simulink model "EKF_SPM_Slx2019"  (R2019a)
settings: Solver=ode45  StartTime=0.0  StopTime=0.7  MaxStep=5e-6  RelTol=1e-3
values from neighbouring files (symbols this model uses):
  alpha = 2*pi*200    (= 1256.63706144)    [EKF_SPM_settings.m]
  alphas = log(9)/t_rc    [EKF_SPM_settings.m]
  d = [-1/Ld; 0]    [EKF_SPM_settings.m]
  fpwm = 20e3    (= 20000)    [EKF_SPM_settings.m]
  gainAngle_noise = 0    [EKF_SPM_settings.m]
  gainSpeed_noise = 3.6 /60*2*pi    (= 0.376991118431)    [EKF_SPM_settings.m]
  inertia = 1.8e-4    (= 0.00018)    [EKF_SPM_settings.m]
  ivar = istdDev^2    (= 11.6508444444)    [EKF_SPM_settings.m]
  J = skewdec(2,0)    [EKF_SPM_settings.m]
  Kbs = 2/Kp_speed    [EKF_SPM_settings.m]
  ki = (-5.135 + 5.347)/Ts    (= 4240)    [EKF_SPM_settings.m]
  Ki_speed = (alphas/2/zeta)^2*inertia    [EKF_SPM_settings.m]
  kp = 5.347    [EKF_SPM_settings.m]
  Kp_speed = alphas*inertia    [EKF_SPM_settings.m]
  Ld = 3e-3    (= 0.003)    [EKF_SPM_settings.m]
  Linv = inv(L)    [EKF_SPM_settings.m]
  Lq = 3e-3    (= 0.003)    [EKF_SPM_settings.m]
  LT = 2.8    [EKF_SPM_settings.m]
  m = 3    [EKF_SPM_settings.m]
  p = 4    [EKF_SPM_settings.m]
  P0 = diag([0.1 0.1 200 10])    [EKF_SPM_settings.m]
  phi_PM = 0.1    [EKF_SPM_settings.m]
  Q = eye(4)    [EKF_SPM_settings.m]
  Qd = eye(4)    [EKF_SPM_settings.m]
  R = 1.9    [EKF_SPM_settings.m]
  R_cov = meas_sd^2*eye(2)    [EKF_SPM_settings.m]
  ramp_rate = 5    [EKF_SPM_settings.m]
  Rs = R    (= 1.9)    [EKF_SPM_settings.m]
  seed_1 = round(rand*(2^32-1))    [EKF_SPM_settings.m]
  seed_2 = round(rand*(2^32-1))    [EKF_SPM_settings.m]
  seed_4 = round(rand*(2^32-1))    [EKF_SPM_settings.m]
  seed_5 = round(rand*(2^32-1))    [EKF_SPM_settings.m]
  seed_6 = round(rand*(2^32-1))    [EKF_SPM_settings.m]
  snoise_mean = 0    [EKF_SPM_settings.m]
  snoise_std = 0.5    [EKF_SPM_settings.m]
  Ts = 1/fpwm    (= 5e-05)    [EKF_SPM_settings.m]
  Tspeed = Ts*10/10    (= 5e-05)    [EKF_SPM_settings.m]
  Vdc = 450    [EKF_SPM_settings.m]
  wm = 2*pi*ff    (= 1675.51608191)    [EKF_SPM_settings.m]
  zeta = 0.9    [EKF_SPM_settings.m]
undefined symbols (not defined in the file or in its folder): ssensor
libraries: simulink x11
(part 2 of 2)

== matlab function EKF_SPM_Slx2019/SUBMOTOR 2/Current_Controller/current control Lane 2 ==
  data: Udc input; id_ref input; iq_ref input; v_alpha output; is input; ws input; thetas input; Ld parameter; Lq parameter; xd input; xq input; v_beta output; xd_new output; xq_new output; alpha parameter; Ts parameter; Rs parameter; measNoise_d input; measNoise_q input; id output; iq output
function [ v_alpha, v_beta, xd_new, xq_new , id, iq] = cc_Lane2(Udc,id_ref,iq_ref,is,ws,thetas,Ld, Lq, xd, xq,alpha, Ts, Rs,measNoise_d, measNoise_q)

if ~iscolumn(is)
    is = is';
end

%% Current controller 

% current split
ialpha = is(1);
ibeta = is(2);

%% angle adjustment for the second motor
% (for the second sub-motor we need to make a shift of pi/6)
% park transform of the feedback
co = cos(thetas);
si = sin(thetas);
id = co*ialpha + si*ibeta;
iq = -si*ialpha + co*ibeta;
% adding noise
id = id + measNoise_d;
iq = iq + measNoise_q;

% compute ideal voltage ref in dq-coordinates
ed = id_ref - id;
eq = iq_ref - iq;
ud = alpha*Ld*ed - ws*Lq*iq + xd;
uq = alpha*Lq*eq + ws*Ld*id + xq;

% Reference in stator coordinates
thetasc = thetas + 1*Ts*ws;   % discrete-time delays
uss_ref = (ud + 1i*uq) * exp(1j*thetasc); % compensation

%% Preparing valpha - vbeta for SVM - with saturation 
% Components of the voltage space vector
ualpha_ref = real(uss_ref);
ubeta_ref  = imag(uss_ref);

% maximum modulation index for the power converter (SVM implementation 
% according to Lee: A novel overmodulation technique for spece vector PWM Inverters)
uss_abs = hypot(ubeta_ref,ualpha_ref);
mi = uss_abs/(2/pi*Udc);

% clamping and building reference in alpha-beta frame
if mi >= 1 
    uss_abs = 2/pi*Udc;
    phase_ref = atan2(ualpha_ref,ubeta_ref);
    uss_ref_lim = uss_abs*(cos(phase_ref) + 1j*sin(phase_ref));
else
    uss_ref_lim = uss_ref;
end

% In estimated rotor flux coordinates
us_ref_lim = exp(-1j*thetasc)*uss_ref_lim; 

% back to real dq
vd = real(us_ref_lim);
vq = imag(us_ref_lim);

%% Back calculate with integration 
xd_new = xd + Ts*Rs/Ld*(vd - xd + ws*Lq*iq);
xq_new = xq + Ts*Rs/Lq*(vq - xq - ws*Ld*id);

%% Final reference is still the v_alpha and v_beta
% SHIFT ENFORCED
%uss_ref_lim = uss_ref_lim*exp(-1j*pi/6);
% alpha beta reference
v_alpha = real(uss_ref_lim);
v_beta = imag(uss_ref_lim);

end

== matlab function EKF_SPM_Slx2019/SUBMOTOR 2/Nicola Chiodetto SVM + Overmodulation ==
  data: v_alpha input; ma output; v_beta input; Vdc input; mb output; mc output; mi output
function [ma,mb,mc,mi] = svm_overmodulation(v_alpha,v_beta,Vdc)
% svm_overmodulation is a matlab-simulink embedded function 
% it implements: 
% - space vector modulation in linear region (within inscribed circle of the hexagon)
% - overmodulation in both non-linear regions identified by Holtz 
% - it ends up in six step value when the reference imposed equates the max
% voltage provided by an inverter leg; namely 2/3*Vdc

% NC @December 2019 - Adjustment July2020

[sector,theta] = sextant(v_alpha,v_beta);   % sector detection

[va,vb,vat, vbt, adj,mi] = overmodulation(v_alpha,v_beta,sector,theta,Vdc); % overmodulation

[ma,mb,mc] = modulation_indexes(va,vb,sector,adj); % modulation index

end


%%-------------------------------------------------------------------------
% function for sextant detection
function [sector,angle] = sextant(v_alpha,v_beta)

	if (v_beta >= 0)
        % sector detection
		if (abs(v_beta) > sqrt(3)*abs(v_alpha))
			sector = 2;
        else		
			if (v_alpha > 0)
				sector = 1;
			else
				sector = 3;
            end
        end
        % angle detection
        angle = atan2(v_beta,v_alpha);
        
    else
        % sector detection
		if (abs(v_beta) > sqrt(3)*abs(v_alpha))
			sector = 5;
        else		
			if (v_alpha > 0)
				sector = 6;
			else
				sector = 4;
            end
        end
        angle = atan2(v_beta,v_alpha)+2*pi;  
    end 
      
end

%--------------------------------------------------------------------------
% function the modulation indexes definition
function [ma,mb,mc] = modulation_indexes(v_alpha,v_beta,sector,adj)

    % added by Nicola Chiodetto @02 October 2020
    mi_lim = 1.0; 

    % assignment
    %mod_idx = zeros(1,3);
    ma = 0;
    mb = 0;
    mc = 0;
    
    ROOT3 = sqrt(3);

	switch sector 
	
		case 1            
            vds = v_alpha;
            vqs = v_beta;
			[ua,ub,uc] = vector_decomposition(vds,vqs,adj);
			ma = ua + ub + uc*0.5;
			mb = ub + uc*0.5;
			mc = 0.5*uc;		           

		case 2            
			% rotate clockwise of 60 deg
			vds = -0.5*v_alpha + ROOT3*0.5*v_beta;
			vqs = ROOT3*0.5*v_alpha + 0.5*v_beta;
			[ua,ub,uc] = vector_decomposition(vds,vqs,adj);
			ma = ub + 0.5*uc;
			mb = ua + ub + 0.5*uc;
			mc = 0.5*uc;           
			
		case 3            
			% rotate clockwise of 120 deg
			vds = -0.5*v_alpha + ROOT3*0.5*v_beta;
			vqs = -ROOT3*0.5*v_alpha - 0.5*v_beta;
			[ua,ub,uc] = vector_decomposition(vds,vqs,adj);
			ma = 0.5*uc;
			mb = ua+ ub + 0.5*uc;
			mc = ub + 0.5*uc;           
                     
		case 4            
			% rotate clockwise of 180 deg
			vds = -0.5*v_alpha - ROOT3*0.5*v_beta;
			vqs = -ROOT3*0.5*v_alpha +0.5*v_beta;
			[ua,ub,uc] = vector_decomposition(vds,vqs,adj);
			ma = 0.5*uc;
			mb = ub + 0.5*uc;
			mc = ua + ub + 0.5*uc;			            
            
		case 5
			% rotating clockwise of 240 deg
			vds = -0.5*v_alpha - ROOT3*0.5*v_beta;
			vqs = ROOT3*0.5*v_alpha - 0.5*v_beta;
			[ua,ub,uc] = vector_decomposition(vds,vqs,adj);
			ma = ub + 0.5*uc;
			mb = 0.5*uc;
			mc = ua + ub + 0.5*uc;
			
		case 6
			% rotating clockwise of 300 deg
			vds = v_alpha;
			vqs = -v_beta;
			[ua,ub,uc] = vector_decomposition(vds,vqs,adj);
			ma = ua + ub + 0.5*uc;
			mb = 0.5*uc;
			mc = ub + 0.5*uc;
            
    end  
    
    % lower saturation
    if ma <= 0; ma = 0;    end
    if mb <= 0; mb = 0;    end
    if mc <= 0; mc = 0;    end
    
    % upper saturation
    if ma >= 1; ma = mi_lim;    end
    if mb >= 1; mb = mi_lim;    end
    if mc >= 1; mc = mi_lim;    end
    
end

%--------------------------------------------------------------------------
% function for vector decomposition along the 2 sector axis
function [ua,ub,uc] = vector_decomposition(v_alpha,v_beta,adjust)

	ub = 2/sqrt(3) * v_beta;
	ua = v_alpha - v_beta/sqrt(3); % 0.5 is equivalent to cos(60)
	uc = 1 - ua - ub;

    % adjustment in case we hit the hexagon
    if (adjust == 1)
        ua_temp = ua;
        ua = ua/(ua+ub);
        ub = ub/(ua_temp+ub);
        uc = 0;
    end
    
end

%--------------------------------------------------------------------------
% function for overmodulation check: it returns the modified voltage
% reference vector in case of overmodulation. It refers already to the
% first sector (so we need to bring back the vector in advance)
function [v_alpha , v_beta, v_alpha_temp, v_beta_temp adj, mi] = overmodulation(v_alpha,v_beta,sector,angle,Vdc)

% assignment
v_alpha_temp = 0;
v_beta_temp = 0;

% init adjustment exception
    adj = 0;

% choose the algorithm to apply (normal or overmodulation scheme)
    mag = hypot(v_alpha,v_beta);
    mi = mag*pi/(2*Vdc);
    
    v_alpha = v_alpha*3/2/Vdc;
    v_beta = v_beta*3/2/Vdc;
    
    % Overmodulation region I *********************************************
    % This is based on Lee : NOVEL OVERMODULATION TECHNIQUE FOR
    % SPACE-VECTOR PWM INVERTERS
        
    if (mi > 0.9068 && mi < 0.9517) 
        
        % reference angle linearization
        if mi < 0.9095
            alpha_r = -30.23*mi + 27.94;     
        elseif mi < 0.9485
                alpha_r = -8.58*mi + 8.23;
        else
            alpha_r = -26.43*mi + 25.15;
        end
        
        % sector angle adjustment
        angle = angle - (sector-1)*pi/3; 
        
        % generating modified reference voltage for the first quadrant
        if angle < alpha_r
            v_alpha_temp = 1/sqrt(3)*1/cos(pi/6-alpha_r)*cos(angle);
            v_beta_temp = 1/sqrt(3)*1/cos(pi/6-alpha_r)*sin(angle);
        elseif angle < pi/3-alpha_r
            v_alpha_temp = 1/sqrt(3)*1/cos(pi/6-angle)*cos(angle);
            v_beta_temp = 1/sqrt(3)*1/cos(pi/6-angle)*sin(angle);
            adj = 1; % along the hexagon enforcement
        elseif angle >= pi/3-alpha_r
            v_alpha_temp = 1/sqrt(3)*1/cos(pi/6-alpha_r)*cos(angle);
            v_beta_temp = 1/sqrt(3)*1/cos(pi/6-alpha_r)*sin(angle);
        else
            %warning('change of sector. you need to implement stuff or is mistake: you should not be here.')
        end       
        
        % final tuning for the sectors (rotating back)      
        v_alpha = cos((sector-1)*pi/3)*v_alpha_temp - sin((sector-1)*pi/3)*v_beta_temp;
        v_beta = sin((sector-1)*pi/3)*v_alpha_temp + cos((sector-1)*pi/3)*v_beta_temp;
        
        adj = 1; % along the hexagon enforcement
        
        return
        
    end    
    %**********************************************************************
    
    % Overmodulation region II*********************************************
    % THIS IS BASED ON HOLTZ: ON CONTINUOUS CONTROL OF PWM INVERTERS IN THE
    % OVEMODULATION RANGE INCLUDING THE SIX STEP MODE
    
    % this overmodulation region works by sector (not quadrant)
    
    if (mi > 0.9517 && mi < 1)
       
        % holding angle linearization
        if mi < 0.98
            alpha_h = 6.4*mi -6.09;     
        elseif mi < 0.9975
                alpha_h = 11.75*mi -11.34;
        else
            alpha_h = 48.96*mi - 48.43;
        end
        
        % angle adjustment depending on sector
        angle = angle - (sector-1)*pi/3;
        
        % phase angle
        if angle < alpha_h
            alpha_p = 0;
        elseif angle < pi/3-alpha_h
            %alpha_p = (angle-alpha_h)/(pi/6-alpha_h)*pi/6;
            alpha_p = angle/(1-3/pi*alpha_h);
        else
            alpha_p = pi/3;
        end
        
        % generating modified reference voltage for the first quadrant
        if angle < alpha_h
            v_alpha_temp = 2/3;
            v_beta_temp = 0;
        elseif angle < pi/3-alpha_h
%             v_alpha_temp = 1/sqrt(3)*1/cos(pi/6-alpha_p)*cos(alpha_p);
%             v_beta_temp = 1/sqrt(3)*1/cos(pi/6-alpha_p)*sin(alpha_p);
            v_alpha_temp = 2/sqrt(3)*1/(tan(alpha_p)+sqrt(3)); 
            v_beta_temp = 2/sqrt(3)*1/(tan(alpha_p)+sqrt(3))*tan(alpha_p);
        elseif angle >= pi/3-alpha_h
            v_alpha_temp = 1/3;
            v_beta_temp = 1/sqrt(3);
        else
            %warning('change of sector. you need to implement stuff or is mistake: you should not be here.')
        end       
        
        % final tuning for the sectors (rotating back)      
        v_alpha = cos((sector-1)*pi/3)*v_alpha_temp - sin((sector-1)*pi/3)*v_beta_temp;
        v_beta = sin((sector-1)*pi/3)*v_alpha_temp + cos((sector-1)*pi/3)*v_beta_temp;
       
        % always along the hexagon enforcement
        adj = 1;
        
        return       
        
    end    
    %**********************************************************************
    
    % Out of space
    if mi > 1.0
       error('Not acceptable modulation index');               
    end
    
end

== matlab function EKF_SPM_Slx2019/Speed_Controller1/Check_AdvancedFF ==
  data: w_ref input; wn_1 input; wn_2 input; w_meas input; I input; Tffn_1 input; Tffn_2 input; Te output; Inew output; Tffn output; Kp_speed parameter; Ki_speed parameter; inertia parameter; zeta parameter; alphas parameter; Tspeed parameter; m parameter; sat output; Kbs parameter
function [ Te, Inew, Tffn, sat ]   = sc_2DOF_advancedff( w_ref, wn_1, wn_2, w_meas, ...
                                                    I, Tffn_1, Tffn_2 , ...
                                                    Kp_speed, Ki_speed, inertia, zeta, alphas, Tspeed, m, Kbs) 

% assignment for concise writing
T = Tspeed;
J = inertia;

% % saturation limit
% P_lim = 2*1.1e3;
% % Extension
% T_lim = P_lim/abs(w_meas);
% % Retraction
T_lim = 15;

%% Torque ref building

T_ref = Kp_speed*(w_ref-w_meas) + Ki_speed*I + Tffn_1;

%% Saturation block

if T_ref >= T_lim
    Te = T_lim;
    sat = 1;
elseif T_ref <= -T_lim
    Te = -T_lim;
    sat = 1;
else
    Te = T_ref;
    sat = 0;
end

%% Integrator + back-calculation antiwindup

Inew = I + Tspeed*(w_ref-w_meas + Kbs*(Te - T_ref));

%% Feedforward

a0 = 1; a1 = 2*m*alphas; a2 = m^2*alphas^2;
b0 = J*alphas*(2*m-1); b1 = J*alphas^2*(m^2-1/zeta^2);

% speed entrance measurement
xn = w_ref;
xn1 = wn_1;
xn2 = wn_2;
% ff signal
yn1 = Tffn_1;
yn2 = Tffn_2;

yn = ((b1*(xn - xn1))/T - a2*yn1 + (a0*(2*yn1 - yn2))/T^2 + (b0*(xn - 2*xn1 + xn2))/T^2 + (a1*yn1)/T)/(a1/T + a0/T^2);
Tffn = yn;

end

== matlab function EKF_SPM_Slx2019/Current ref building1/IPM ==
  data: Tref input; id output; iq output; Imag output
function [id, iq, Imag] = ipm_current_refence( Tref )
% pre-made functions (analytical linear) current reference build up

% coefficients for the cubic interpolation (current vs torque)
cd = [0.0033
   -0.0283
    0.5322
   -0.0407];
cq = [-0.0041
    5.4017
   -0.0449
   -0.0221];

% id
id = cd(1) + Tref*cd(2) + Tref^2*cd(3) + Tref^3*cd(4);
% iq
iq = cq(1) + Tref*cq(2) + Tref^2*cq(3) + Tref^3*cq(4);

% magnitude
Imag = hypot(id,iq);

end

== matlab function EKF_SPM_Slx2019/Current ref building1/SPM-current reference ==
  data: T_ref input; id output; phi_PM parameter; p parameter; iq output; Imag output
function [id, iq, Imag] = spm_current_refence( T_ref, phi_PM, p)

% ideal-analytical-MTPA
if abs(T_ref) < 1e-5
    iq = 0;
else
    iq = T_ref/(1.5*phi_PM*p);
end

id = 0;

Imag = hypot(id,iq);

end

== matlab function EKF_SPM_Slx2019/1 DOF controller ==
  data: w_ref input; w_meas input; Te output; Inew output; Iw input; Ki_speed parameter; Kp_speed parameter; Tspeed parameter
function [Te,Inew] = PI_1DOF(w_ref,w_meas,Iw, Ki_speed, Kp_speed, Tspeed)
% recycled routine from the current controller

%Tspeed = Ts*10;

%% error
ew = w_ref - w_meas;

%% PI controller
T_ref = Kp_speed*ew + Ki_speed*Iw;    % prop

%% ANTI WINDUP SATURATION
T_lim = 4;

% Saturation block

if T_ref >= T_lim
    Te = T_lim;
    sat = 1;
elseif T_ref <= -T_lim
    Te = -T_lim;
    sat = 1;
else
    Te = T_ref;
    sat = 0;
end

Inew = Iw + Tspeed*(ew + 2/Kp_speed*(Te - T_ref));

end

== matlab function EKF_SPM_Slx2019/SUBMOTOR 2/HealthySUbmotor - PI//1/Adding current system noise1/MATLAB Function ==
  data: mean input; y output; stdDev input; s1 input
function y  = white_gauss_noise(mean,stdDev,s1)

% NC generation of gauss white noise with the simulation period (not sampling period)

% defining the seed of interest for this simulation
persistent first_fcn_call
if isempty(first_fcn_call)
    rand('seed',s1);
    first_fcn_call = 0;
end

spare = 0;
hasSpare = 0;

if(hasSpare)
    hasSpare = 0;
    y = spare*stdDev + mean;
else
    % init var for loops
    s = 0; u = 0; v = 0;
    while(s >= 1.0 || s == 0)
        u = rand * 2.0 - 1.0;
        v = rand * 2.0 - 1.0;        
        s = u^2+v^2;
    end
    s = sqrt(-2.0*log(s)/s);
    spare = v*s;
    hasSpare = 1;
    y = mean + stdDev*u*s;
end

== matlab function EKF_SPM_Slx2019/SUBMOTOR 2/Current_Controller/Emulate Measurement noise on dq axis/MATLAB Function1 ==
  data: mean input; y output; stdDev input; s1 input
function y  = white_gauss_noise(mean,stdDev,s1)

% NC generation of gauss white noise with the simulation period (not sampling period)

% defining the seed of interest for this simulation
persistent first_fcn_call
if isempty(first_fcn_call)
    rand('seed',s1);
    first_fcn_call = 0;
end

spare = 0;
hasSpare = 0;

if(hasSpare)
    hasSpare = 0;
    y = spare*stdDev + mean;
else
    % init var for loops
    s = 0; u = 0; v = 0;
    while(s >= 1.0 || s == 0)
        u = rand * 2.0 - 1.0;
        v = rand * 2.0 - 1.0;        
        s = u^2+v^2;
    end
    s = sqrt(-2.0*log(s)/s);
    spare = v*s;
    hasSpare = 1;
    y = mean + stdDev*u*s;
end

== matlab function EKF_SPM_Slx2019/SUBMOTOR 2/HealthySUbmotor - PI//1/Adding current system noise1/MATLAB Function2 ==
  data: mean input; y output; stdDev input; s2 input
function y  = white_gauss_noise(mean,stdDev,s2)

% NC generation of gauss white noise with the simulation period (not sampling period)

persistent first_fcn_call
if isempty(first_fcn_call)
    rand('seed',s2);
    first_fcn_call = 0;
end

spare = 0;
hasSpare = 0;

if(hasSpare)
    hasSpare = 0;
    y = spare*stdDev + mean;
else
    % init var for loops
    s = 0; u = 0; v = 0;
    while(s >= 1.0 || s == 0)
        u = rand * 2.0 - 1.0;
        v = rand * 2.0 - 1.0;        
        s = u^2+v^2;
    end
    s = sqrt(-2.0*log(s)/s);
    spare = v*s;
    hasSpare = 1;
    y = mean + stdDev*u*s;
end

== matlab function EKF_SPM_Slx2019/limit 0 - 360 ==
  data: u input; y output
function y = adjust_angle(u)

% keep it bounded in its true range
while (u >= 2*pi)
    u = u - 2*pi;
end

y = u;

== matlab function EKF_SPM_Slx2019/SUBMOTOR 2/Emulate Measurement noise on dq axis/MATLAB Function ==
  data: mean input; y output; stdDev input; s1 input
function y  = white_gauss_noise(mean,stdDev,s1)

% NC generation of gauss white noise with the simulation period (not sampling period)

% defining the seed of interest for this simulation
persistent first_fcn_call
if isempty(first_fcn_call)
    rand('seed',s1);
    first_fcn_call = 0;
end

spare = 0;
hasSpare = 0;

if(hasSpare)
    hasSpare = 0;
    y = spare*stdDev + mean;
else
    % init var for loops
    s = 0; u = 0; v = 0;
    while(s >= 1.0 || s == 0)
        u = rand * 2.0 - 1.0;
        v = rand * 2.0 - 1.0;        
        s = u^2+v^2;
    end
    s = sqrt(-2.0*log(s)/s);
    spare = v*s;
    hasSpare = 1;
    y = mean + stdDev*u*s;
end

== matlab function EKF_SPM_Slx2019/SUBMOTOR 2/Emulate Measurement noise on dq axis/MATLAB Function1 ==
  data: mean input; y output; stdDev input; s1 input
function y  = white_gauss_noise(mean,stdDev,s1)

% NC generation of gauss white noise with the simulation period (not sampling period)

% defining the seed of interest for this simulation
persistent first_fcn_call
if isempty(first_fcn_call)
    rand('seed',s1);
    first_fcn_call = 0;
end

spare = 0;
hasSpare = 0;

if(hasSpare)
    hasSpare = 0;
    y = spare*stdDev + mean;
else
    % init var for loops
    s = 0; u = 0; v = 0;
    while(s >= 1.0 || s == 0)
        u = rand * 2.0 - 1.0;
        v = rand * 2.0 - 1.0;        
        s = u^2+v^2;
    end
    s = sqrt(-2.0*log(s)/s);
    spare = v*s;
    hasSpare = 1;
    y = mean + stdDev*u*s;
end

== matlab function EKF_SPM_Slx2019/MATLAB Function ==
  data: u input; y output
function y = trace(u)


y = sum(diag(u));

== matlab function EKF_SPM_Slx2019/SUBMOTOR 2/Emulate Measurement noise on dq axis1/MATLAB Function ==
  data: mean input; y output; stdDev input; s1 input
function y  = white_gauss_noise(mean,stdDev,s1)

% NC generation of gauss white noise with the simulation period (not sampling period)

% defining the seed of interest for this simulation
persistent first_fcn_call
if isempty(first_fcn_call)
    rand('seed',s1);
    first_fcn_call = 0;
end

spare = 0;
hasSpare = 0;

if(hasSpare)
    hasSpare = 0;
    y = spare*stdDev + mean;
else
    % init var for loops
    s = 0; u = 0; v = 0;
    while(s >= 1.0 || s == 0)
        u = rand * 2.0 - 1.0;
        v = rand * 2.0 - 1.0;        
        s = u^2+v^2;
    end
    s = sqrt(-2.0*log(s)/s);
    spare = v*s;
    hasSpare = 1;
    y = mean + stdDev*u*s;
end

== matlab function EKF_SPM_Slx2019/SUBMOTOR 2/Emulate Measurement noise on dq axis1/MATLAB Function1 ==
  data: mean input; y output; stdDev input; s1 input
function y  = white_gauss_noise(mean,stdDev,s1)

% NC generation of gauss white noise with the simulation period (not sampling period)

% defining the seed of interest for this simulation
persistent first_fcn_call
if isempty(first_fcn_call)
    rand('seed',s1);
    first_fcn_call = 0;
end

spare = 0;
hasSpare = 0;

if(hasSpare)
    hasSpare = 0;
    y = spare*stdDev + mean;
else
    % init var for loops
    s = 0; u = 0; v = 0;
    while(s >= 1.0 || s == 0)
        u = rand * 2.0 - 1.0;
        v = rand * 2.0 - 1.0;        
        s = u^2+v^2;
    end
    s = sqrt(-2.0*log(s)/s);
    spare = v*s;
    hasSpare = 1;
    y = mean + stdDev*u*s;
end

== matlab function EKF_SPM_Slx2019/Get updated Q PSD ==
  data: C input; y output; K input; y_priori output
function [y,y_priori] = adaptive_bit(C,K)

y_priori = K*C*K';

%% Nearest PSDS Matrix Algorithm

% Step 1: Construct the symmetric B matrix, and skew−symmetric C matrix
B = (y_priori + y_priori')/2;
%C = (A − A')/2; %(Not needed for calculations)

% Step 2: Compute the symmetric polar factor of B
[U,Sigma,V] = svd(B);
H = V*Sigma*V';

% Step 3: Compute the positive approximant matrix, symmetricize
A_hat = (B+H)/2;
A_hat = (A_hat + A_hat')/2;

% % Step 4: Testing for PSD, adjusting A_hat if not
% p = 1;
% k = 0;
% while p ~= 0
%     [~,p] = chol(A_hat);
%     %Restrict number of iterations
%     k = k + 1;
%     if k > 5
%         fprintf('Forced break after 5 iterations \n')
%     break
%     end
% 
%     %If A_hat is not PSDS, perturb it a bit
%     if p ~= 0
%         min_eig = 0;
%         min_eig = min(eig(A_hat));
% 
%         A_hat = A_hat + (-min_eig*k.^2 + eps(min_eig))*eye(size(A));
%     end
% end

y = A_hat; % spitting out result
